simulink subsystem "Outer_loop"  (R2024a)
settings: Solver=VariableStepAuto  StartTime=0.0  StopTime=10.0  RelTol=1e-3
settings Model: Creator=gurt1  LastModifiedBy=gurt1
settings RTWCC: GPUComputeCapability=3.5

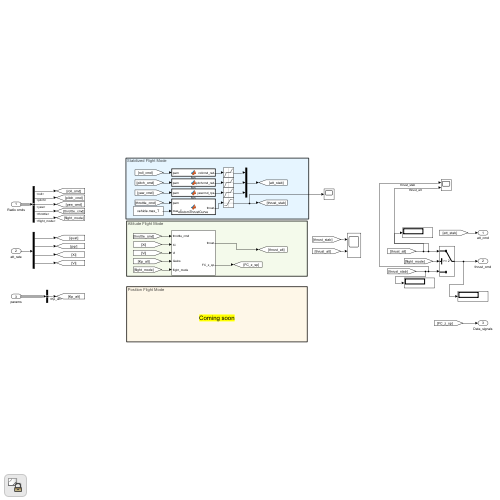
[thumbnail: Simulink's stored preview of the top-level diagram]
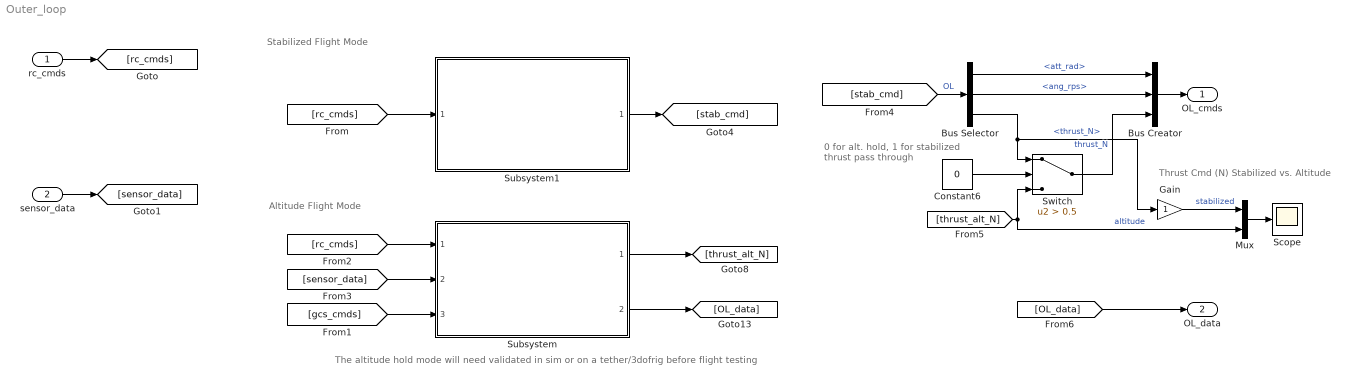
== system Outer_loop ==
  note: Thrust Cmd (N) Stabilized vs. Altitude
  note: 0 for alt. hold, 1 for stabilized thrust pass through
  note: The altitude hold mode will need validated in sim or on a tether/3dofrig before flight testing
  note: Altitude Flight Mode
  note: Stabilized Flight Mode
  rc_cmds : Inport
  sensor_data : Inport  Port=2
  Bus Creator : BusCreator  Inputs=3
  Bus Selector : BusSelector  OutputSignals=att_rad,ang_rps,thrust_N
  Constant6 : Constant  Value=0
  Gain : Gain
  Mux : Mux  Inputs=2
  Scope : Scope
  Subsystem : Subsystem  ReferencedSubsystem=Altitude
  Subsystem1 : Subsystem  ReferencedSubsystem=Stabilized
  Switch : Switch  Criteria=u2 > Threshold  Threshold=0.5  SaturateOnIntegerOverflow=off  InputSameDT=off
  OL_cmds : Outport
  OL_data : Outport  Port=2
  wires:
  sensor_data/1 -> [sensor_data]
  Subsystem/1 -> [thrust_alt_N]
  [rc_cmds] -> Subsystem/1
  [sensor_data] -> Subsystem/2
  [gcs_cmds] -> Subsystem/3
  Subsystem/2 -> [OL_data]
  rc_cmds/1 -> [rc_cmds]
  [rc_cmds] -> Subsystem1/1
  Subsystem1/1 -> [stab_cmd]
  [OL_data] -> OL_data/1
  [stab_cmd] -> Bus Selector/1  "OL"
  Bus Selector/3 -> Switch/1, Gain/1  "<thrust_N>"
  [thrust_alt_N] -> Mux/2, Switch/3  "altitude"
  Bus Creator/1 -> OL_cmds/1
  Bus Selector/1 -> Bus Creator/1  "<att_rad>"
  Bus Selector/2 -> Bus Creator/2  "<ang_rps>"
  Switch/1 -> Bus Creator/3  "thrust_N"
  Constant6/1 -> Switch/2
  Mux/1 -> Scope/1
  Gain/1 -> Mux/1  "stabilized"
